simulink model "Full_Adder_2_Bit"  (R2020a)
settings: Solver=VariableStepAuto  StartTime=0.0  StopTime=10.0  RelTol=1e-3
settings Model: Creator=ashwin  LastModifiedBy=ashwin

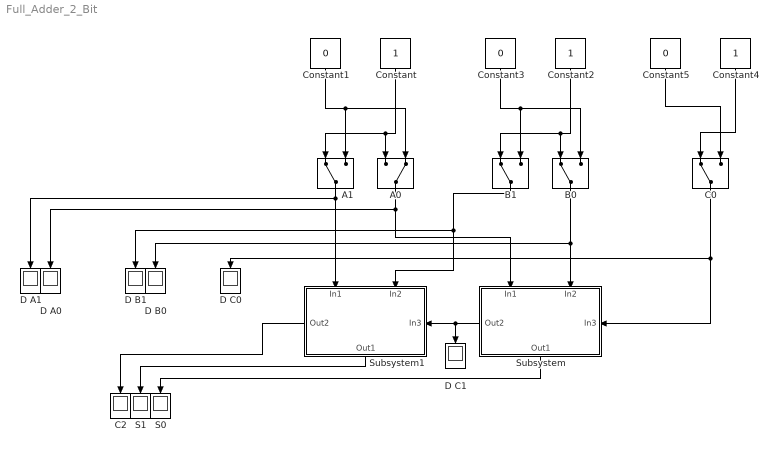
== system Full_Adder_2_Bit ==
  A0 : ManualSwitch  CurrentSetting=0
  A1 : ManualSwitch
  B0 : ManualSwitch
  B1 : ManualSwitch
  C0 : ManualSwitch
  C2 : Display
  Constant : Constant
  Constant1 : Constant  Value=0
  Constant2 : Constant
  Constant3 : Constant  Value=0
  Constant4 : Constant
  Constant5 : Constant  Value=0
  D A0 : Display
  D A1 : Display
  D B0 : Display
  D B1 : Display
  D C0 : Display
  D C1 : Display
  S0 : Display
  S1 : Display
  Subsystem : Subsystem
      settings: PortSchema="{\"entries\":[{\"content\":{\"sides\":[{\"content\":{\"connectorIds\":[\"In1\",\"In2\"]},\"type\":\"ConnectorPlacement.EquallySpacedRectSide\",\"uuid\":\"2a5ccbd8-a607-4e8e-aeab-6573d843420d\"},{\"content\":{\"connectorIds\":[\"Out1\"],\"side\":\"RIGHT\"},\"type\":\"ConnectorPlacement.EquallySpacedRectSide\",\"uuid\":\"6267f48a-d68e-44d4-8735-4b8fc9221377\"},{\"content\":{\"connectorIds\":[\"Out2\"],\"side\":\"TOP\"},\"type\":\"ConnectorPlacement.EquallySpacedRectSide\",\"uuid\":\"3feafea9-4ba3-4cfb-8323-0c0a7fedf83d\"},{\"content\":{\"connectorIds\":[\"In3\"],\"side\":\"BOTTOM\"},\"type\":\"ConnectorPlacement.EquallySpacedRectSide\",\"uuid\":\"727fb993-98ee-44f6-b335-4a395a1676fd\"}]},\"type\":\"ConnectorPlacement.EquallySpacedConnector\",\"uuid\":\"13fcee94-3465-4beb-9827-9174468a15e8\"}],\"packageUris\":[\"http://schema.mathworks.com/mf0/Connector/19700101\"],\"version\":\"1.0\"}"
      mask Display:
      | disp('1-bit FA');
      | 
      | port_label('input', 1, 'A');
      | port_label('input', 2, 'B');
      | port_label('input', 3, 'Ci');
      | 
      | port_label('output', 1, 'S');
      | port_label('output', 2, 'Co');
  Subsystem1 : Subsystem
      settings: PortSchema="{\"entries\":[{\"content\":{\"sides\":[{\"content\":{\"connectorIds\":[\"In1\",\"In2\"]},\"type\":\"ConnectorPlacement.EquallySpacedRectSide\",\"uuid\":\"2a5ccbd8-a607-4e8e-aeab-6573d843420d\"},{\"content\":{\"connectorIds\":[\"Out1\"],\"side\":\"RIGHT\"},\"type\":\"ConnectorPlacement.EquallySpacedRectSide\",\"uuid\":\"6267f48a-d68e-44d4-8735-4b8fc9221377\"},{\"content\":{\"connectorIds\":[\"Out2\"],\"side\":\"TOP\"},\"type\":\"ConnectorPlacement.EquallySpacedRectSide\",\"uuid\":\"3feafea9-4ba3-4cfb-8323-0c0a7fedf83d\"},{\"content\":{\"connectorIds\":[\"In3\"],\"side\":\"BOTTOM\"},\"type\":\"ConnectorPlacement.EquallySpacedRectSide\",\"uuid\":\"727fb993-98ee-44f6-b335-4a395a1676fd\"}]},\"type\":\"ConnectorPlacement.EquallySpacedConnector\",\"uuid\":\"13fcee94-3465-4beb-9827-9174468a15e8\"}],\"packageUris\":[\"http://schema.mathworks.com/mf0/Connector/19700101\"],\"version\":\"1.0\"}"
      mask Display:
      | disp('1-bit FA');
      | 
      | port_label('input', 1, 'A');
      | port_label('input', 2, 'B');
      | port_label('input', 3, 'Ci');
      | 
      | port_label('output', 1, 'S');
      | port_label('output', 2, 'Co');
  wires:
  Subsystem/2(Out2) -> D C1/1, Subsystem1/3(In3)
  Subsystem1/2(Out2) -> C2/1
  Subsystem1/1(Out1) -> S1/1
  Subsystem/1(Out1) -> S0/1
  Constant1/1 -> A0/2, A1/2
  Constant/1 -> A1/1, A0/1
  Constant2/1 -> B1/1, B0/1
  Constant3/1 -> B1/2, B0/2
  Constant5/1 -> C0/2
  Constant4/1 -> C0/1
  C0/1 -> D C0/1, Subsystem/3(In3)
  A1/1 -> D A1/1, Subsystem1/1(In1)
  A0/1 -> D A0/1, Subsystem/1(In1)
  B1/1 -> D B1/1, Subsystem1/2(In2)
  B0/1 -> D B0/1, Subsystem/2(In2)

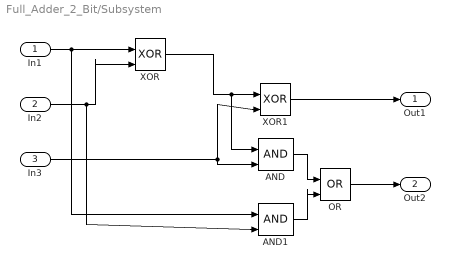
== system Full_Adder_2_Bit/Subsystem ==
  In1 : Inport
  In2 : Inport  Port=2
  In3 : Inport  Port=3
  AND : Logic  IconShape=distinctive  AllPortsSameDT=off  OutDataTypeStr=boolean
  AND1 : Logic  IconShape=distinctive  AllPortsSameDT=off  OutDataTypeStr=boolean
  OR : Logic  Operator=OR  IconShape=distinctive  AllPortsSameDT=off  OutDataTypeStr=boolean
  XOR : Logic  Operator=XOR  IconShape=distinctive  AllPortsSameDT=off  OutDataTypeStr=boolean
  XOR1 : Logic  Operator=XOR  IconShape=distinctive  AllPortsSameDT=off  OutDataTypeStr=boolean
  Out1 : Outport
  Out2 : Outport  Port=2
  wires:
  OR/1 -> Out2/1
  XOR1/1 -> Out1/1
  AND1/1 -> OR/2
  AND/1 -> OR/1
  In3/1 -> XOR1/2, AND/2
  XOR/1 -> AND/1, XOR1/1
  In1/1 -> AND1/1, XOR/1
  In2/1 -> AND1/2, XOR/2

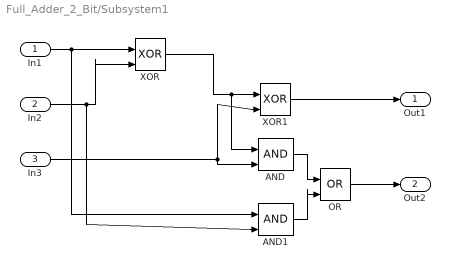
== system Full_Adder_2_Bit/Subsystem1 ==
  In1 : Inport
  In2 : Inport  Port=2
  In3 : Inport  Port=3
  AND : Logic  IconShape=distinctive  AllPortsSameDT=off  OutDataTypeStr=boolean
  AND1 : Logic  IconShape=distinctive  AllPortsSameDT=off  OutDataTypeStr=boolean
  OR : Logic  Operator=OR  IconShape=distinctive  AllPortsSameDT=off  OutDataTypeStr=boolean
  XOR : Logic  Operator=XOR  IconShape=distinctive  AllPortsSameDT=off  OutDataTypeStr=boolean
  XOR1 : Logic  Operator=XOR  IconShape=distinctive  AllPortsSameDT=off  OutDataTypeStr=boolean
  Out1 : Outport
  Out2 : Outport  Port=2
  wires:
  OR/1 -> Out2/1
  XOR1/1 -> Out1/1
  AND1/1 -> OR/2
  AND/1 -> OR/1
  In3/1 -> XOR1/2, AND/2
  XOR/1 -> AND/1, XOR1/1
  In1/1 -> AND1/1, XOR/1
  In2/1 -> AND1/2, XOR/2
